simulink model "QtrCarPassive"  (R2013a)
settings: Solver=ode23s  StartTime=0.0  StopTime=tfin  FixedStep=0.0001  RelTol=1e-5
undefined symbols (not defined in the file or in its folder): a, Ac, amp, Ap, Cb, Ci, Ck, cp, Cts, Ctus, cv, dx, dy, g, gamma, initial, Jm, lambda1, lambda2, lambda3, meq, ms, mus, OnOff, P0, P10, Pcrit, R, rm, Rw, sigbuilder_block, T, tau, U, V10, wnf, x, y, zeta_pas
settings Model: Creator=Layne  LastModifiedBy=Iceman
settings DataIOCC: SignalLoggingSaveFormat=ModelDataLogs
settings DebuggingCC: AlgebraicLoopMsg=none  UnderspecifiedInitializationDetection=Simplified  MultiTaskDSMMsg=warning  MultiTaskCondExecSysMsg=none  StateNameClashWarn=none  StrictBusMsg=ErrorOnBusTreatedAsVector
settings RTWCC: IncludeERTFirstTime=on
settings GRTTargetCC: CodeReplacementLibrary=None  CPPClassGenCompliant=on

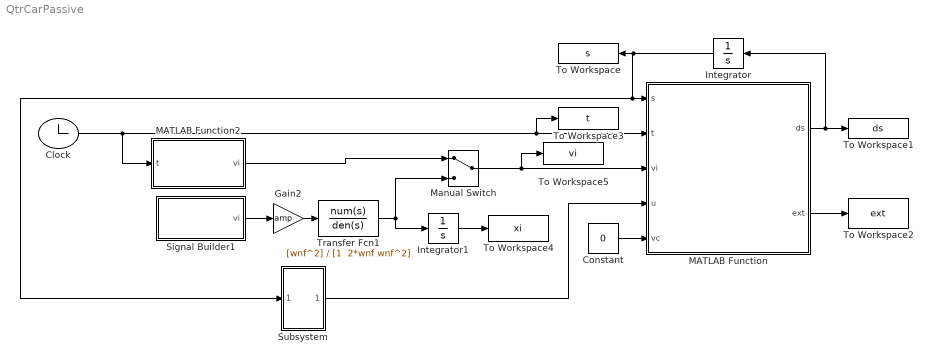
== system QtrCarPassive ==
  Clock : Clock
  Constant : Constant  Value=0
  Gain2 : Gain  Gain=amp
  Integrator : Integrator  InitialCondition=initial
  Integrator1 : Integrator
  MATLAB Function : MATLAB Function  TreatAsAtomicUnit=on
  MATLAB Function2 : MATLAB Function  TreatAsAtomicUnit=on
  Manual Switch : ManualSwitch
  Signal Builder1 : Subsystem  Tag=STV Subsys  LoadFcn=sigbuilder_block('load');  StartFcn=sigbuilder_block('start');  StopFcn=sigbuilder_block('stop');  ClipboardFcn=sigbuilder_block('clipboard');  mask(Sigbuilder block){}
      mask help: Simulink:masks:SigbuilderBlock_MD
      mask init:
      | if ~strcmp(get_param(bdroot(gcbh),'SimulationStatus'),'stopped') tuvar = sigbuilder_block('maskInit'); end
      settings: CopyFcn=sigbuilder_block('copy');  DeleteFcn=sigbuilder_block('delete');  ModelCloseFcn=sigbuilder_block('modelClose');  PreSaveFcn=sigbuilder_block('preSave');  PauseFcn=sigbuilder_block('pause');  ContinueFcn=sigbuilder_block('continue');  NameChangeFcn=sigbuilder_block('namechange');  OpenFcn=sigbuilder_block('open',[266.25 144 544.5 391.5 ]);  CloseFcn=sigbuilder_block('close');
      mask Display: plot(0, 0, 100, 100,[2, 2, 32, 32, 2], [68, 8, 8, 68, 68],[32, 2], [38, 38], [32, 19, 2],[53, 60, 44], [32, 17, 17, 2],[16, 16, 31, 31]);txt = getActiveGroup(gcbh);text(2, 100, txt,'verticalAlignment', 'top');
  Subsystem : Subsystem
  To Workspace : ToWorkspace  VariableName=s  SampleTime=-1
  To Workspace1 : ToWorkspace  VariableName=ds  SampleTime=-1
  To Workspace2 : ToWorkspace  VariableName=ext  SampleTime=-1
  To Workspace3 : ToWorkspace  VariableName=t  SampleTime=-1
  To Workspace4 : ToWorkspace  VariableName=xi  SampleTime=-1
  To Workspace5 : ToWorkspace  VariableName=vi  SampleTime=-1
  Transfer Fcn1 : TransferFcn  Numerator=[wnf^2]  Denominator="[1  2*wnf wnf^2]"
  wires:
  MATLAB Function/1(ds) -> Integrator/1, To Workspace1/1
  Clock/1 -> MATLAB Function2/1(t), To Workspace3/1, MATLAB Function/2(t)
  MATLAB Function/2(ext) -> To Workspace2/1
  Integrator/1 -> Subsystem/1(In1), MATLAB Function/1(s), To Workspace/1
  Constant/1 -> MATLAB Function/5(vc)
  Subsystem/1(Out1) -> MATLAB Function/4(u)
  Signal Builder1/1(vi) -> Gain2/1
  Gain2/1 -> Transfer Fcn1/1
  Transfer Fcn1/1 -> Manual Switch/2, Integrator1/1
  Integrator1/1 -> To Workspace4/1
  Manual Switch/1 -> To Workspace5/1, MATLAB Function/3(vi)
  MATLAB Function2/1(vi) -> Manual Switch/1

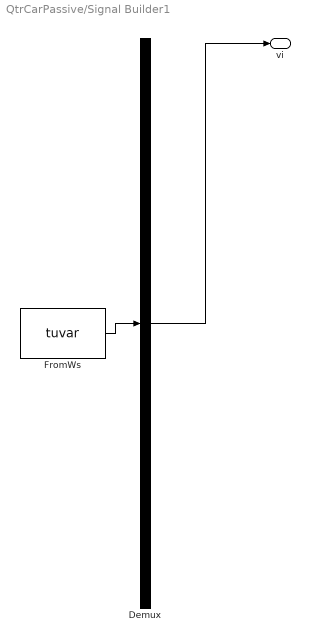
== system QtrCarPassive/Signal Builder1 ==
  Demux : Demux  Tag=STV Demux  Outputs=1
  FromWs : FromWorkspace  Tag=STV FromWs  VariableName=tuvar  SampleTime=0
      SigBuilderData=|
      | common.afterFinalStr = 'Extrapolate'
      | common.sampleTime = 0
      | dataSet.timeRange = [0 10]
      | dataSet.name = 'Group 1'
      | sbobj.Groups.Name = 'Group 1'
      | sbobj.Groups.Signals.Name = 'vi'
      | sbobj.Groups.Signals.XData = [0 1 1 1.0136 1.0136 1.0272 1.0272 10]
      | sbobj.Groups.Signals.YData = [0 0 1 1 -1 -1 0 0]
  vi : Outport  Tag=STV Outport
  wires:
  Demux/1 -> vi/1
  FromWs/1 -> Demux/1

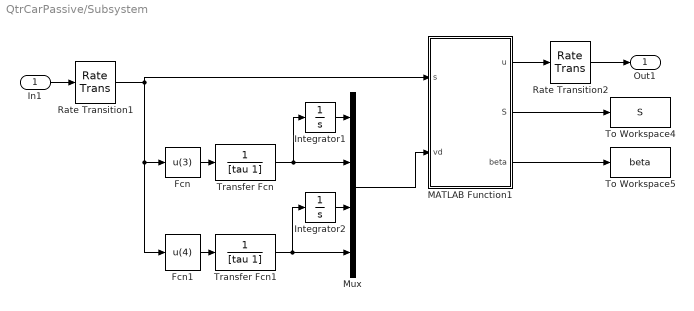
== system QtrCarPassive/Subsystem ==
  In1 : Inport
  Fcn : Fcn  Expr=u(3)
  Fcn1 : Fcn  Expr=u(4)
  Integrator1 : Integrator
  Integrator2 : Integrator
  MATLAB Function1 : MATLAB Function  TreatAsAtomicUnit=on
  Mux : Mux
  Rate Transition1 : RateTransition  OutPortSampleTime=Ts
  Rate Transition2 : RateTransition
  To Workspace4 : ToWorkspace  VariableName=S  SampleTime=-1
  To Workspace5 : ToWorkspace  VariableName=beta  SampleTime=-1
  Transfer Fcn : TransferFcn  Denominator=[tau 1]
  Transfer Fcn1 : TransferFcn  Denominator=[tau 1]
  Out1 : Outport
  wires:
  MATLAB Function1/2(S) -> To Workspace4/1
  MATLAB Function1/3(beta) -> To Workspace5/1
  Fcn/1 -> Transfer Fcn/1
  Fcn1/1 -> Transfer Fcn1/1
  Integrator2/1 -> Mux/3
  Transfer Fcn/1 -> Integrator1/1, Mux/2
  Transfer Fcn1/1 -> Integrator2/1, Mux/4
  Integrator1/1 -> Mux/1
  MATLAB Function1/1(u) -> Rate Transition2/1
  Mux/1 -> MATLAB Function1/2(vd)
  In1/1 -> Rate Transition1/1
  Rate Transition1/1 -> MATLAB Function1/1(s), Fcn1/1, Fcn/1
  Rate Transition2/1 -> Out1/1

== matlab function QtrCarPassive/MATLAB Function ==
  data: s input; t input; vi input; u input; vc input; ds output; Ctus parameter; Cts parameter; Ck parameter; Cb parameter; Ci parameter; ext output; mus parameter; ms parameter; OnOff parameter; meq parameter; a parameter; cp parameter; cv parameter; R parameter; Ap parameter; Ac parameter; gamma parameter; Pcrit parameter; P0 parameter; Jm parameter; rm parameter; g parameter; T parameter; Rw parameter
function [ds,ext] = QtrCar(s,t,vi,u,vc,Ctus,Cts,Ck,Cb,Ci,mus,ms,OnOff,meq,a,cp,cv,R,Ap,Ac,gamma,Pcrit,P0,Jm,rm,g,T,Rw)

% Unpack the state vector. The state vector has been augmented with 2 free
% integrators which integrate vs and vus for control.
qt = s(1);
vus = s(2);
vs = s(3);
V1 = s(4);
V2 = s(5);
E1 = s(6);
E2 = s(7);
m1 = s(8);
m2 = s(9);
vus_i = s(10);
vs_i = s(11);
qs = s(12);

ic = OnOff*u(1);
vc = 0;
% vi = 0;
%% Calculate internal variables needed in equations
P1 = R*E1/(cv*V1);
P2 = R*E2/(cv*V2);
T1 = E1/(cv*m1);
T2 = E2/(cv*m2);
Fk = Ap*(P1-P0);
% if t > 1 && t < 1.1
%     vc = 0;
% end
% if abs(vc) < 10^-3
%     vc = 0;
% end
if V1 > 1.5*3.8E-3
    vc = 0 ;
end

if V1 < 0.5*3.8E-3
    vc = 0 ;
end
%% Calculate energy and mass flows through the thermodynamic resistor
% Find the upstream and downstream pressures 
if P1 >= P2
    Pu = P1;
    Pd = P2;
    Tu = T1;
else
    Pu = P2;
    Pd = P1;
    Tu = T2;
end

% Calculate the reduced pressure
Pr = Pd/Pu;
if Pr <= Pcrit
    Pr = Pcrit;
end
% Pd
% Pu
% Pr
% sqrt(Pr^(2/gamma)-Pr^((gamma+1)/gamma))
% sqrt(2*gamma/(R*(gamma-1)))
% Calculate the mass flow rate
if abs(vc)>10^-1
   d0=1*0.7*0.0254;
else
   d0=0;
end
A0 = pi*d0^2/4;
mdot = A0*Pu/sqrt(abs(Tu))*sqrt(abs(2*gamma/(R*(gamma-1))))*sqrt(abs(Pr^(2/gamma)-Pr^((gamma+1)/gamma)));

% set the mass flows
if P1 > P2
    mdot_a = mdot;
    mdot_b = mdot;
else
    mdot_a = -mdot;
    mdot_b = -mdot;
end

% Calculate the energy flow
% Tu = 1;
% mdot_a =0;
% mdot_b = 0;
Edot_a = cp*Tu*mdot_a;
Edot_b = cp*Tu*mdot_a;


%% Calculate the state time derivatives
ds = zeros(12,1);
ds(1) = vi - vus;
ds(2) = 1/mus*(Ctus*qt - Cb*vus + Cb*vs - 1/a*Fk - Ci*ic...
        -(Jm+ms*rm^2)/(a*ms*rm^2)*mus*g - Jm/(a*rm^2)*g);
ds(3) = 1/ms*(Cts*qt + 1/a*Fk + Cb*vus - Cb*vs + Ci*ic...
        -(Jm+mus*rm^2)/(a*mus*rm^2)*ms*g - Jm/(a*rm^2)*g);
ds(4) = -Ac*vc-Ap*(vus-vs);
ds(5) = Ac*vc;
ds(6) = -Edot_a - P1*ds(4);
ds(7) = Edot_b - P2*ds(5);
ds(8) = -mdot_a;
ds(9) = mdot_b;
ds(10) = vus;
ds(11) = vs;
ds(12) = vus-vs;
ds;
ext = zeros(4,1);
ext(1) = ic;
ext(2) = P1;
ext(3) = P2;
ext(4) = vc;
% ext(4)
P = T/rm*ic*(vus-vs)-Rw*ic^2;
vrel = vus-vs;
Pv = [P1,P2];

== matlab function QtrCarPassive/MATLAB Function2 ==
  data: vi output; t input; dx parameter; dy parameter; x parameter; y parameter; U parameter
function vi  = roadInput(t,dx,dy,x,y,U)
% Unpack the state vector
xt = U*t;
i = floor(xt/dx);
vi = U*dy(i+1)/dx;

== matlab function QtrCarPassive/Subsystem/MATLAB Function1 ==
  data: s input; vd input; ms parameter; Ap parameter; gamma parameter; P10 parameter; P0 parameter; V10 parameter; u output; S output; rm parameter; T parameter; zeta_pas parameter; lambda1 parameter; lambda2 parameter; lambda3 parameter; beta output; a parameter
function [u,S,beta] = controller(s,vd,ms,Ap,gamma,P10,P0,V10,rm,T,zeta_pas,lambda1,lambda2,lambda3,a)
% Unpack the state vector
qt = s(1);
vus = s(2);
vs = s(3);
V1 = s(4);
V2 = s(5);
E1 = s(6);
E2 = s(7);
m1 = s(8);
m2 = s(9);
vus_i = s(10);
vs_i = s(11);
qs = s(12);

vusi_d = vd(1);
vus_d = vd(2);
vsi_d = vd(3);
vs_d = vd(4);
% ks = s(7);
% Calculate each surface
S1 = (vs-vs_d) + lambda1*(vs_i-vsi_d);
S2 = (vus-vus_d) + lambda2*(vus_i-vusi_d);
S3 = vus-vs + lambda3*qs;
S = [S1;S2;S3];
% Control parameters
u = 2*a*rm*Ap*sqrt(gamma*(P10-P0)*ms)*zeta_pas/(T*sqrt(V10))*(vus-vs);
beta = 0;
